simulink model "LidarSLAMIn3DSimulation"  (R2024b)
settings: Solver=VariableStepAuto  StartTime=0.0  StopTime=106.1385  RelTol=1e-3
PreLoadFcn:
  | % Load reference path for recorded drive segment
  | xData   = load('refPosesX.mat');
  | yData   = load('refPosesY.mat');
  | yawData = load('refPosesT.mat');
  | 
  | % Set up workspace variables used by model
  | refPosesX = xData.refPosesX;
  | refPosesY = yData.refPosesY;
  | refPosesT = yawData.refPosesT;
  | 
  | % Load INS measurement
  | insMeasurement = load('insMeasurement.mat');
  | insMeasurement = insMeasurement.insMeasurement;
undefined symbols (not defined in the file or in its folder): Sim3dSensor
libraries: sim3dphyssensorlib x3, sim3dautolib x3, sim3dlib x1
settings Model: Creator=The MathWorks, Inc.  LastModifiedBy=yashk
settings SolverCC: AlgebraicLoopSolver=TrustRegion
settings DebuggingCC: UnconnectedInputMsg=warning  UnconnectedOutputMsg=warning  UnconnectedLineMsg=warning  SymbolicDimsDataTypeCodeGenerationDiagnostic=none
settings ModelReferenceCC: EnableRefExpFcnMdlSchedulingChecks=on
settings RTWCC: GPUComputeCapability=3.5

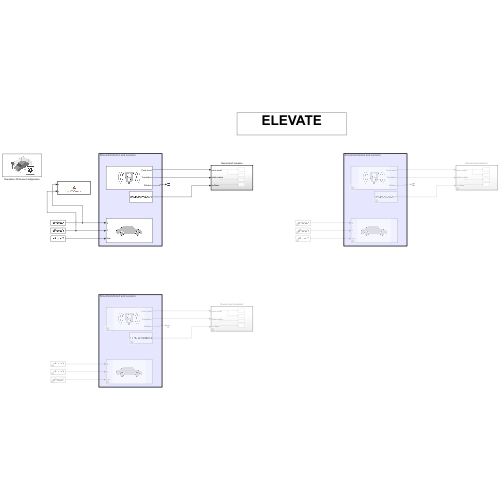
[thumbnail: Simulink's stored preview of the top-level diagram]
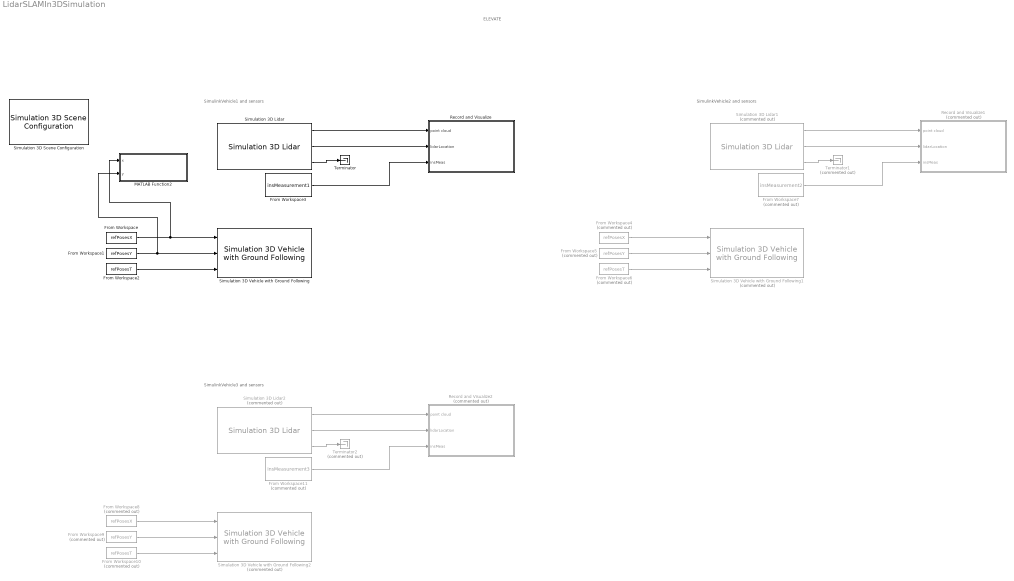
== system LidarSLAMIn3DSimulation ==
  note: ELEVATE
  note: SimulinkVehicle1 and sensors
  note: SimulinkVehicle2 and sensors
  note: SimulinkVehicle3 and sensors
  From Workspace : FromWorkspace  VariableName=refPosesX  OutputAfterFinalValue=Holding final value
  From Workspace1 : FromWorkspace  VariableName=refPosesY  OutputAfterFinalValue=Holding final value
  From Workspace10 : FromWorkspace  Commented=on  VariableName=refPosesT  Interpolate=off  OutputAfterFinalValue=Holding final value
  From Workspace11 : FromWorkspace  Commented=on  VariableName=insMeasurement3  SampleTime=0.1  Interpolate=off  OutputAfterFinalValue=Holding final value
  From Workspace2 : FromWorkspace  VariableName=refPosesT  Interpolate=off  OutputAfterFinalValue=Holding final value
  From Workspace3 : FromWorkspace  VariableName=insMeasurement1  SampleTime=0.1  Interpolate=off  OutputAfterFinalValue=Holding final value
  From Workspace4 : FromWorkspace  Commented=on  VariableName=refPosesX  OutputAfterFinalValue=Holding final value
  From Workspace5 : FromWorkspace  Commented=on  VariableName=refPosesY  OutputAfterFinalValue=Holding final value
  From Workspace6 : FromWorkspace  Commented=on  VariableName=refPosesT  Interpolate=off  OutputAfterFinalValue=Holding final value
  From Workspace7 : FromWorkspace  Commented=on  VariableName=insMeasurement2  SampleTime=0.1  Interpolate=off  OutputAfterFinalValue=Holding final value
  From Workspace8 : FromWorkspace  Commented=on  VariableName=refPosesX  OutputAfterFinalValue=Holding final value
  From Workspace9 : FromWorkspace  Commented=on  VariableName=refPosesY  OutputAfterFinalValue=Holding final value
  MATLAB Function2 : MATLAB Function  TreatAsAtomicUnit=on
      settings: ModelCloseFcn=|
      | % Find figure with name "Scene Display"
      | hFig = findobj('Type', 'figure', 'Name', 'Scene Display');
      | 
      | if ~isempty(hFig) && isvalid(hFig)
      |     close(hFig);
      | end
      | clear hFig;
  Record and Visualize : Subsystem  TreatAsAtomicUnit=on
  Record and Visualize1 : Subsystem  Commented=on  TreatAsAtomicUnit=on
  Record and Visualize2 : Subsystem  Commented=on  TreatAsAtomicUnit=on
  Simulation 3D Lidar : sim3dphyssensorlib/Simulation 3D Lidar  sensorTag=Sim3dSensor�  sensorId=1  sensorName=Sim3dSensor�  vehTagList={'Scene Origin';'SimulinkVehicle1';'SimulinkVehicle2';'SimulinkVehicle3'}  vehTag=SimulinkVehicle1  mountLoc=Roof center  offsetFlag=off  tmountOffset=[0, 0, 0]  rmountOffset=[0, 0, 0]  DetectionRange=90  RangeResolution=0.002  VerticalFOV=40  VerticalResolution=1.25  HorizontalFOV=360  HorizontalResolution=0.332409972299169  DistanceOutportEnabled=off  ReflectivityOutportEnabled=off  SemanticOutportEnabled=off  TransformOutportEnabled=on  SampleTime=0.1  mountPoint=[-0.45 0 1.68]  mountOrientation=[0 0 0]  aMode=3  ID=1
      settings: LibrarySourceBlock=drivingsim3d/Simulation 3D Lidar
  Simulation 3D Lidar1 : sim3dphyssensorlib/Simulation 3D Lidar  Commented=on  sensorTag=Sim3dSensor�  sensorId=2  sensorName=Sim3dSensor�  vehTagList={'Scene Origin';'SimulinkVehicle1';'SimulinkVehicle2';'SimulinkVehicle3'}  vehTag=SimulinkVehicle2  mountLoc=Front bumper  offsetFlag=off  tmountOffset=[0, 0, 0]  rmountOffset=[0, 0, 0]  DetectionRange=90  RangeResolution=0.002  VerticalFOV=40  VerticalResolution=1.25  HorizontalFOV=360  HorizontalResolution=0.332409972299169  DistanceOutportEnabled=off  ReflectivityOutportEnabled=off  SemanticOutportEnabled=off  TransformOutportEnabled=on  SampleTime=0.1  mountPoint=[2.424 0 0.5]  mountOrientation=[0 0 0]  aMode=3  ID=2
      settings: LibrarySourceBlock=drivingsim3d/Simulation 3D Lidar
  Simulation 3D Lidar2 : sim3dphyssensorlib/Simulation 3D Lidar  Commented=on  sensorTag=Sim3dSensor�  sensorId=3  sensorName=Sim3dSensor�  vehTagList={'Scene Origin';'SimulinkVehicle1';'SimulinkVehicle2';'SimulinkVehicle3'}  vehTag=SimulinkVehicle3  mountLoc=Hood center  offsetFlag=off  tmountOffset=[0, 0, 0]  rmountOffset=[0, 0, 0]  DetectionRange=90  RangeResolution=0.002  VerticalFOV=40  VerticalResolution=1.25  HorizontalFOV=360  HorizontalResolution=0.332409972299169  DistanceOutportEnabled=off  ReflectivityOutportEnabled=off  SemanticOutportEnabled=off  TransformOutportEnabled=on  SampleTime=0.1  mountPoint=[1.464 0 1.1]  mountOrientation=[0 0 0]  aMode=3  ID=3
      settings: LibrarySourceBlock=drivingsim3d/Simulation 3D Lidar
  Simulation 3D Scene Configuration : sim3dlib/Simulation 3D Scene Configuration  Priority=0  ProjectFormat=Default Scenes  SceneDesc=US city block  ProjectName=C:\Program Files\MATLAB\R2024b\toolbox\shared\sim3d_projects\automotive_project_windows\UE\WindowsNoEditor\VehicleSimulation.exe  ScenePath=/Game/Maps/HwStrght  EnableOpenDRIVE=off  vehTagList={'Custom';'Scene Origin';'SimulinkVehicle1';'SimulinkVehicle2';'SimulinkVehicle3'}  vehTag=SimulinkVehicle1  FreeCameraInitialTranslation=[0, 0, 0]  FreeCameraDefaultInitialTranslation=[-6, 0, 2]  FreeCameraInitialRotation=[0, 0, 0]  FreeCameraDefaultInitialRotation=[0, -15, 0]  OpVisEn=off  Ts=0.1  EnableWindow=on  EnableRemoteAccess=off  EnableWeather=off  SunAzimuth=90  SunAltitude=40.0  EnableGeospatialSun=off  Latitude=0  Longitude=0  Date=2023-01-01  Time=10:30:00  GeoTimeZone=-5.0  SunDaylightSaving=off  wind=1  clouds=10  EnableVolumetricClouds=off  CloudCoverage=0  CloudAltitude=6  fog=0  rain=0  RaindropsEffect=off  SnowDensity=0  EnableGeospatial=off  UseTrueOrigin=off  OriginHeight=200  OriginLatitude=40.744652  OriginLongitude=-73.988864  MapStyle=Aerial  AdditionalAssetIDs=[]  UseAdvancedSunSky=off  SolarTime=11  TimeZone=-5  Day=21  Month=9  Year=2022  UseDaylightSavingTime=on  DSTStartDay=10  DSTStartMonth=3  DSTEndDay=3  DSTEndMonth=11  DSTSwitchHour=2  sensorTag=MainCamera1  sensorId=1  sensorName=MainCamera1  mountLoc=Origin  offsetFlag=off  tmountOffset=[0, 0, 0]  rmountOffset=[0, 0, 0]  HorizontalResolution=1280  VerticalResolution=720  HorizontalFOV=60  mountPoint=[0 0 0]  mountOrientation=[0 0 0]  aMode=3  ID=1  GeoTrigger=Inactive
      settings: LibrarySourceBlock=drivingsim3d/Simulation 3D Scene Configuration
  Simulation 3D Vehicle with Ground Following : sim3dautolib/Simulation 3D Vehicle with Ground Following  Priority=-1  PassVehMesh=Sedan  MeshPath=/MathWorksAutomotiveContent/Vehicles/Muscle/Meshes/SK_MuscleCar.SK_MuscleCar  TrackWidth=1.9  WheelBase=3  WheelRadius=0.35  VehColor=Silver  InitialPos=[refPosesX(1,2), refPosesY(1,2), 0]  InitialRot=[0, 0, refPosesT(1,2)]  ActorName=SimulinkVehicle1  SampleTime=-1  ActorType=SimulinkVehicle  ID=1  aMode=3  ActorTag=SimulinkVehicle1  CoordinateScheme=ISO  VehLightsControl=off  HeadlightColor=[ 1, 1, 1 ]  HighBeamIntensity=100000  LowBeamIntensity=60000  HighBeamConeAngle=70  LowBeamConeAngle=70  LeftHeadlightOrientation=[ 0, 0 ]  RightHeadlightOrientation=[ 0, 0 ]  BrakelightIntensity=500  ReverselightIntensity=500  SignallightIntensity=500  SignallightPeriod=1  SignalPulseWidth=50  TransformOutportEnabled=off
      settings: LibrarySourceBlock=drivingsim3d/Simulation 3D Vehicle with Ground Following
  Simulation 3D Vehicle with Ground Following1 : sim3dautolib/Simulation 3D Vehicle with Ground Following  Priority=-1  Commented=on  PassVehMesh=Sport utility vehicle  MeshPath=/MathWorksAutomotiveContent/Vehicles/Muscle/Meshes/SK_MuscleCar.SK_MuscleCar  TrackWidth=1.9  WheelBase=3  WheelRadius=0.35  VehColor=Blue  InitialPos=[refPosesX(2,1), refPosesY(2,1), 0]  InitialRot=[0, 0, refPosesT(1,2)]  ActorName=SimulinkVehicle2  SampleTime=-1  ActorType=SimulinkVehicle  ID=2  aMode=3  ActorTag=SimulinkVehicle2  CoordinateScheme=ISO  VehLightsControl=off  HeadlightColor=[ 1, 1, 1 ]  HighBeamIntensity=100000  LowBeamIntensity=60000  HighBeamConeAngle=70  LowBeamConeAngle=70  LeftHeadlightOrientation=[ 0, 0 ]  RightHeadlightOrientation=[ 0, 0 ]  BrakelightIntensity=500  ReverselightIntensity=500  SignallightIntensity=500  SignallightPeriod=1  SignalPulseWidth=50  TransformOutportEnabled=off
      settings: LibrarySourceBlock=drivingsim3d/Simulation 3D Vehicle with Ground Following
  Simulation 3D Vehicle with Ground Following2 : sim3dautolib/Simulation 3D Vehicle with Ground Following  Priority=-1  Commented=on  PassVehMesh=Sedan  MeshPath=/MathWorksAutomotiveContent/Vehicles/Muscle/Meshes/SK_MuscleCar.SK_MuscleCar  TrackWidth=1.9  WheelBase=3  WheelRadius=0.35  VehColor=Silver  InitialPos=[refPosesX(1,1), refPosesY(1,1), 0]  InitialRot=[0, 0, refPosesT(1,2)]  ActorName=SimulinkVehicle3  SampleTime=-1  ActorType=SimulinkVehicle  ID=3  aMode=3  ActorTag=SimulinkVehicle3  CoordinateScheme=ISO  VehLightsControl=off  HeadlightColor=[ 1, 1, 1 ]  HighBeamIntensity=100000  LowBeamIntensity=60000  HighBeamConeAngle=70  LowBeamConeAngle=70  LeftHeadlightOrientation=[ 0, 0 ]  RightHeadlightOrientation=[ 0, 0 ]  BrakelightIntensity=500  ReverselightIntensity=500  SignallightIntensity=500  SignallightPeriod=1  SignalPulseWidth=50  TransformOutportEnabled=off
      settings: LibrarySourceBlock=drivingsim3d/Simulation 3D Vehicle with Ground Following
  Terminator : Terminator
  Terminator1 : Terminator  Commented=on
  Terminator2 : Terminator  Commented=on
  wires:
  From Workspace2/1 -> Simulation 3D Vehicle with Ground Following/3
  Simulation 3D Lidar/1 -> Record and Visualize/1(point cloud)
  From Workspace3/1 -> Record and Visualize/3(insMeas)
  Simulation 3D Lidar/2 -> Record and Visualize/2(lidarLocation)
  Simulation 3D Lidar/3 -> Terminator/1
  Simulation 3D Lidar1/1 -> Record and Visualize1/1(point cloud)
  From Workspace7/1 -> Record and Visualize1/3(insMeas)
  Simulation 3D Lidar1/2 -> Record and Visualize1/2(lidarLocation)
  Simulation 3D Lidar1/3 -> Terminator1/1
  From Workspace5/1 -> Simulation 3D Vehicle with Ground Following1/2
  From Workspace6/1 -> Simulation 3D Vehicle with Ground Following1/3
  From Workspace4/1 -> Simulation 3D Vehicle with Ground Following1/1
  From Workspace10/1 -> Simulation 3D Vehicle with Ground Following2/3
  Simulation 3D Lidar2/3 -> Terminator2/1
  From Workspace11/1 -> Record and Visualize2/3(insMeas)
  Simulation 3D Lidar2/2 -> Record and Visualize2/2(lidarLocation)
  From Workspace9/1 -> Simulation 3D Vehicle with Ground Following2/2
  Simulation 3D Lidar2/1 -> Record and Visualize2/1(point cloud)
  From Workspace8/1 -> Simulation 3D Vehicle with Ground Following2/1
  From Workspace1/1 -> MATLAB Function2/2(y), Simulation 3D Vehicle with Ground Following/2
  From Workspace/1 -> MATLAB Function2/1(x), Simulation 3D Vehicle with Ground Following/1

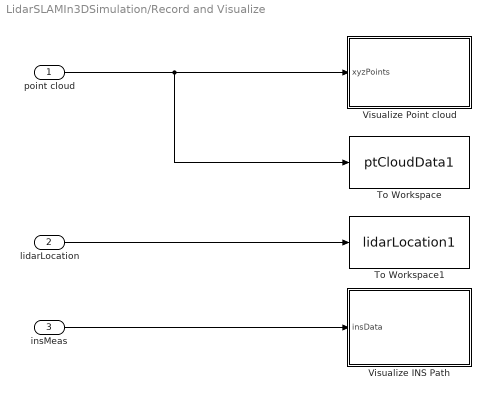
== system LidarSLAMIn3DSimulation/Record and Visualize ==
  point cloud : Inport
  lidarLocation : Inport  Port=2
  insMeas : Inport  Port=3
  To Workspace : ToWorkspace  VariableName=ptCloudData1  SaveFormat=Structure With Time  SampleTime=-1
  To Workspace1 : ToWorkspace  VariableName=lidarLocation1  SaveFormat=Structure With Time  SampleTime=-1
  Visualize INS Path : MATLAB Function  StopFcn=|  TreatAsAtomicUnit=on
      | playerFigure = findall(groot,'type','figure','name','INS Sensor Display');
      | 
      | if ~isempty(playerFigure)
      |     playerFigure = playerFigure(end);
      |     if isvalid(playerFigure)
      |         close(playerFigure);
      |     end
      | end
  Visualize Point cloud : MATLAB Function  StopFcn=|  TreatAsAtomicUnit=on
      | playerFigure = findall(groot,'type','figure','name','Point Cloud Player');
      | 
      | if ~isempty(playerFigure)
      |     playerFigure = playerFigure(end);
      |     if isvalid(playerFigure)
      |         close(playerFigure);
      |     end
      | end
  wires:
  point cloud/1 -> To Workspace/1, Visualize Point cloud/1(xyzPoints)
  insMeas/1 -> Visualize INS Path/1(insData)
  lidarLocation/1 -> To Workspace1/1

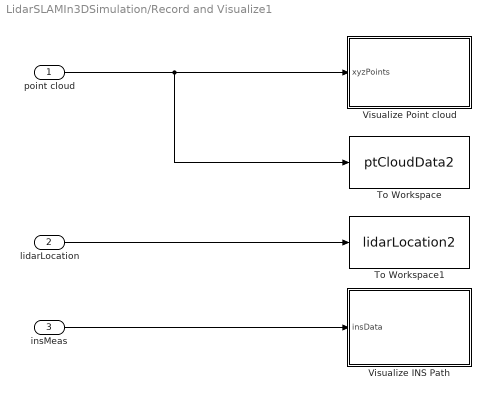
== system LidarSLAMIn3DSimulation/Record and Visualize1 ==
  point cloud : Inport
  lidarLocation : Inport  Port=2
  insMeas : Inport  Port=3
  To Workspace : ToWorkspace  VariableName=ptCloudData2  SaveFormat=Structure With Time  SampleTime=-1
  To Workspace1 : ToWorkspace  VariableName=lidarLocation2  SaveFormat=Structure With Time  SampleTime=-1
  Visualize INS Path : MATLAB Function  StopFcn=|  TreatAsAtomicUnit=on
      | playerFigure = findall(groot,'type','figure','name','INS Sensor Display');
      | 
      | if ~isempty(playerFigure)
      |     playerFigure = playerFigure(end);
      |     if isvalid(playerFigure)
      |         close(playerFigure);
      |     end
      | end
  Visualize Point cloud : MATLAB Function  StopFcn=|  TreatAsAtomicUnit=on
      | playerFigure = findall(groot,'type','figure','name','Point Cloud Player');
      | 
      | if ~isempty(playerFigure)
      |     playerFigure = playerFigure(end);
      |     if isvalid(playerFigure)
      |         close(playerFigure);
      |     end
      | end
  wires:
  insMeas/1 -> Visualize INS Path/1(insData)
  lidarLocation/1 -> To Workspace1/1
  point cloud/1 -> To Workspace/1, Visualize Point cloud/1(xyzPoints)

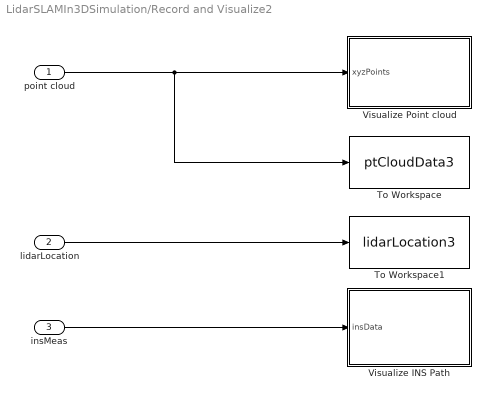
== system LidarSLAMIn3DSimulation/Record and Visualize2 ==
  point cloud : Inport
  lidarLocation : Inport  Port=2
  insMeas : Inport  Port=3
  To Workspace : ToWorkspace  VariableName=ptCloudData3  SaveFormat=Structure With Time  SampleTime=-1
  To Workspace1 : ToWorkspace  VariableName=lidarLocation3  SaveFormat=Structure With Time  SampleTime=-1
  Visualize INS Path : MATLAB Function  StopFcn=|  TreatAsAtomicUnit=on
      | playerFigure = findall(groot,'type','figure','name','INS Sensor Display');
      | 
      | if ~isempty(playerFigure)
      |     playerFigure = playerFigure(end);
      |     if isvalid(playerFigure)
      |         close(playerFigure);
      |     end
      | end
  Visualize Point cloud : MATLAB Function  StopFcn=|  TreatAsAtomicUnit=on
      | playerFigure = findall(groot,'type','figure','name','Point Cloud Player');
      | 
      | if ~isempty(playerFigure)
      |     playerFigure = playerFigure(end);
      |     if isvalid(playerFigure)
      |         close(playerFigure);
      |     end
      | end
  wires:
  point cloud/1 -> To Workspace/1, Visualize Point cloud/1(xyzPoints)
  insMeas/1 -> Visualize INS Path/1(insData)
  lidarLocation/1 -> To Workspace1/1

== matlab function LidarSLAMIn3DSimulation/Record and Visualize1/Visualize INS Path ==
  data: insData input
function visualizeINSPath(insData)
%visualizeINSPath Visualize INS path on scene image
%   helperPlotPath plots the path specified by x,y waypoint on the current
%   scene.

% Copyright 2019 The MathWorks, Inc.

coder.extrinsic('helperShowSceneImage', 'figure', 'title', 'movegui', ...
    'isvalid', 'images.roi.Polyline', 'helperUpdatePolyline', 'xlim', 'ylim');

persistent hFig hPoly;

x = insData(1);
y = insData(2);

bufferZone = [30 30];

if isempty(hFig)
    % Query the model to find the scene selection
    sceneName = 'USCityBlock';
    
    % Create a figure and display the scene on it
    hFig = figure('Name', 'INS Sensor Display');
    helperShowSceneImage(sceneName);
    title('INS Sensor Display');
    
    % Move figure to right of screen
    movegui(hFig, 'east')
    
    % Display the path
    hold on
    hPoly = images.roi.Polyline('Parent', gca, 'Position', [x y], 'InteractionsAllowed', 'none');
end

if isvalid(hFig)
    % Update the path with the new point
    helperUpdatePolyline(hPoly, x, y);
    
    xlims = x + bufferZone(1)*[-1 1];
    ylims = y + bufferZone(2)*[-1 1];
    xlim(xlims);
    ylim(ylims);
end
end

== matlab function LidarSLAMIn3DSimulation/Record and Visualize/Visualize Point cloud ==
  data: xyzPoints input
function VisualizePointCloud(xyzPoints)
%VisualizePointCloud Display point cloud

coder.extrinsic('isOpen', 'pcplayer')

persistent player;

if isempty(player)
    % Configure axes limits
    xlimits = [-90 90];
    ylimits = [-90 90];
    zlimits = [ -5 40];
    
    % Create a streaming Lidar viewer
    player = pcplayer(xlimits, ylimits, zlimits);
end

if ~isempty(player) && isOpen(player)
    view(player, xyzPoints);
end

== matlab function LidarSLAMIn3DSimulation/Record and Visualize/Visualize INS Path ==
  data: insData input
function visualizeINSPath(insData)
%visualizeINSPath Visualize INS path on scene image
%   helperPlotPath plots the path specified by x,y waypoint on the current
%   scene.

% Copyright 2019 The MathWorks, Inc.

coder.extrinsic('helperShowSceneImage', 'figure', 'title', 'movegui', ...
    'isvalid', 'images.roi.Polyline', 'helperUpdatePolyline', 'xlim', 'ylim');

persistent hFig hPoly;

x = insData(1);
y = insData(2);

bufferZone = [30 30];

if isempty(hFig)
    % Query the model to find the scene selection
    sceneName = 'USCityBlock';
    
    % Create a figure and display the scene on it
    hFig = figure('Name', 'INS Sensor Display');
    helperShowSceneImage(sceneName);
    title('INS Sensor Display');
    
    % Move figure to right of screen
    movegui(hFig, 'east')
    
    % Display the path
    hold on
    hPoly = images.roi.Polyline('Parent', gca, 'Position', [x y], 'InteractionsAllowed', 'none');
end

if isvalid(hFig)
    % Update the path with the new point
    helperUpdatePolyline(hPoly, x, y);
    
    xlims = x + bufferZone(1)*[-1 1];
    ylims = y + bufferZone(2)*[-1 1];
    xlim(xlims);
    ylim(ylims);
end
end

== matlab function LidarSLAMIn3DSimulation/Record and Visualize1/Visualize Point cloud ==
  data: xyzPoints input
function VisualizePointCloud(xyzPoints)
%VisualizePointCloud Display point cloud

coder.extrinsic('isOpen', 'pcplayer')

persistent player;

if isempty(player)
    % Configure axes limits
    xlimits = [-90 90];
    ylimits = [-90 90];
    zlimits = [ -5 40];
    
    % Create a streaming Lidar viewer
    player = pcplayer(xlimits, ylimits, zlimits);
end

if ~isempty(player) && isOpen(player)
    view(player, xyzPoints);
end

== matlab function LidarSLAMIn3DSimulation/Record and Visualize2/Visualize INS Path ==
  data: insData input
function visualizeINSPath(insData)
%visualizeINSPath Visualize INS path on scene image
%   helperPlotPath plots the path specified by x,y waypoint on the current
%   scene.

% Copyright 2019 The MathWorks, Inc.

coder.extrinsic('helperShowSceneImage', 'figure', 'title', 'movegui', ...
    'isvalid', 'images.roi.Polyline', 'helperUpdatePolyline', 'xlim', 'ylim');

persistent hFig hPoly;

x = insData(1);
y = insData(2);

bufferZone = [30 30];

if isempty(hFig)
    % Query the model to find the scene selection
    sceneName = 'USCityBlock';
    
    % Create a figure and display the scene on it
    hFig = figure('Name', 'INS Sensor Display');
    helperShowSceneImage(sceneName);
    title('INS Sensor Display');
    
    % Move figure to right of screen
    movegui(hFig, 'east')
    
    % Display the path
    hold on
    hPoly = images.roi.Polyline('Parent', gca, 'Position', [x y], 'InteractionsAllowed', 'none');
end

if isvalid(hFig)
    % Update the path with the new point
    helperUpdatePolyline(hPoly, x, y);
    
    xlims = x + bufferZone(1)*[-1 1];
    ylims = y + bufferZone(2)*[-1 1];
    xlim(xlims);
    ylim(ylims);
end
end

== matlab function LidarSLAMIn3DSimulation/Record and Visualize2/Visualize Point cloud ==
  data: xyzPoints input
function VisualizePointCloud(xyzPoints)
%VisualizePointCloud Display point cloud

coder.extrinsic('isOpen', 'pcplayer')

persistent player;

if isempty(player)
    % Configure axes limits
    xlimits = [-90 90];
    ylimits = [-90 90];
    zlimits = [ -5 40];
    
    % Create a streaming Lidar viewer
    player = pcplayer(xlimits, ylimits, zlimits);
end

if ~isempty(player) && isOpen(player)
    view(player, xyzPoints);
end

== matlab function LidarSLAMIn3DSimulation/MATLAB Function2 ==
  settings: updateMethod=DISCRETE  sampleTime=.02
  data: x input; y input
function plotEVStatus(x, y)
    % Define Simulation Time
    totalTime = 100; % Total simulation time in minutes
    time = linspace(0, totalTime, 100); % Time vector
    
    % Simulate Battery Drain (Linear Decline with Noise)
    initialBattery = 100; % Start at 100%
    batteryLevel = max(0, initialBattery - (time / totalTime) * 100 + randn(size(time)) * 2);
    
    % Simulate Grid Power Levels (Random)
    gridPower = 50 + 20 * randn(size(time)); % Mean at 50% with random fluctuation
    
    % Define Charging Station Locations (Example Data)
    chargers = [10, 20; 30, 50; 60, 40; 90, 80]; % Charging station positions (X, Y)
    vehiclePos = [x, y]; % User-provided vehicle position
    
    % Find Nearest Charger
    distances = vecnorm(chargers - vehiclePos, 2, 2);
    [~, idx] = min(distances);
    nearestCharger = chargers(idx, :);
    
    % Persistent figure and plot handles
    persistent hFig hBattery hGrid hMap hCharger hDistance;

    if isempty(hFig)

        % Create Figure (Only Once)
        hFig = figure('Name', 'EV Data Visualization', 'NumberTitle', 'off');
        
        % Subplot 1: Battery Level Over Time
        subplot(4,1,1);
        hBattery = plot(time, batteryLevel, 'r', 'LineWidth', 2);
        xlabel('Time (min)');
        ylabel('Battery (%)');
        title('Battery Level');
        ylim([0 100]);
        grid on;
        
        % Subplot 2: Grid Power Levels
        subplot(4,1,2);
        hGrid = plot(time, gridPower, 'b', 'LineWidth', 2);
        xlabel('Time (min)');
        ylabel('Grid Power (%)');
        title('Grid Power Availability');
        ylim([0 100]);
        grid on;
        
        % Subplot 3: Vehicle Location & Charger
        subplot(4,1,3);
        hold on;
        hMap = scatter(chargers(:,1), chargers(:,2), 100, 'g', 'filled'); % Chargers
        hCharger = scatter(nearestCharger(1), nearestCharger(2), 200, 'b', 'filled'); % Nearest charger
        scatter(vehiclePos(1), vehiclePos(2), 100, 'r', 'filled'); % Vehicle position
        legend('Charging Stations', 'Nearest Charger', 'Vehicle Position', 'Location', 'Best');
        xlabel('X Position');
        ylabel('Y Position');
        title('Charging Stations');
        grid on;
        
        % Subplot 4: Distance to Nearest Charger Over Time
        subplot(4,1,4);
        hDistance = plot(time, distances(idx) * ones(size(time)), 'k', 'LineWidth', 2);
        xlabel('Time (min)');
        ylabel('Distance (units)');
        title('Distance to Nearest Charger');
        ylim([0 max(distances) + 10]);
        grid on;
    else
        % Update plots instead of creating a new figure
        set(hBattery, 'YData', batteryLevel);
        set(hGrid, 'YData', gridPower);
        set(hCharger, 'XData', nearestCharger(1), 'YData', nearestCharger(2));
        set(hDistance, 'YData', distances(idx) * ones(size(time)));
        drawnow; % Force immediate update
    end
end
